simulink model "exp_2_v2019b"  (R2019b)
settings: Solver=VariableStepAuto  StartTime=0.0  StopTime=10.0  RelTol=1e-3
settings Model: Creator=DELL  LastModifiedBy=DELL

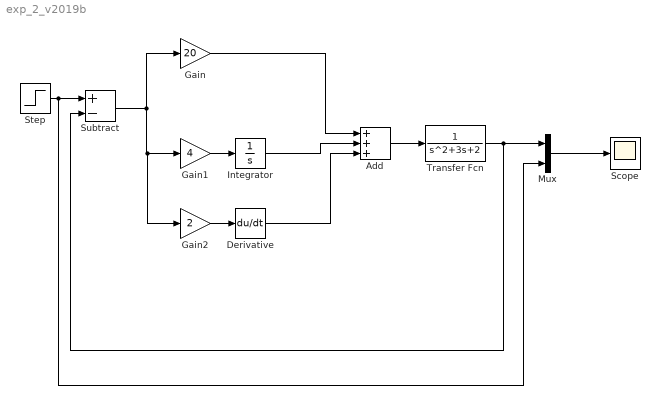
== system exp_2_v2019b ==
  Add : Sum  Inputs=+++
  Derivative : Derivative
  Gain : Gain  Gain=20
  Gain1 : Gain  Gain=4
  Gain2 : Gain  Gain=2
  Integrator : Integrator
  Mux : Mux  Inputs=2
  Scope : Scope
  Step : Step  SampleTime=0
  Subtract : Sum  Inputs=+-
  Transfer Fcn : TransferFcn  Denominator=[1 3 2]
  wires:
  Step/1 -> Subtract/1, Mux/2
  Subtract/1 -> Gain/1, Gain2/1, Gain1/1
  Gain1/1 -> Integrator/1
  Gain2/1 -> Derivative/1
  Gain/1 -> Add/1
  Integrator/1 -> Add/2
  Derivative/1 -> Add/3
  Add/1 -> Transfer Fcn/1
  Mux/1 -> Scope/1
  Transfer Fcn/1 -> Subtract/2, Mux/1
